simulink model "sf_multiword_fixpt"  (R2017b)
settings: Solver=FixedStepDiscrete  StartTime=0.0  StopTime=10.0  RelTol=1e-3  EnableMultiTasking=on
libraries: simulink x1
settings Model: Creator=The MathWorks, Inc.  LastModifiedBy=The MathWorks, Inc.
settings DataIOCC: LimitDataPoints=on  SaveFormat=Array
settings OptimizationCC: ExpressionDepthLimit=2147483647  LifeSpan=inf
settings DebuggingCC: UnderspecifiedInitializationDetection=Classic  MergeDetectMultiDrivingBlocksExec=none  FcnCallInpInsideContextMsg=warning  StateNameClashWarn=warning  StrictBusMsg=Warning  SFUnexpectedBacktrackingDiag=warning  SFNoUnconditionalDefaultTransitionDiag=warning  SFExecutionAtInitializationDiag=none
settings HardwareCC: ProdBitPerLong=64  ProdBitPerPointer=32  ProdBitPerSizeT=32  ProdBitPerPtrDiffT=32  ProdLargestAtomicFloat=None  ProdIntDivRoundTo=Undefined  ProdEndianess=Unspecified  ProdWordSize=32  ProdHWDeviceType=Generic->Custom  TargetHWDeviceType=32-bit Generic
settings ModelReferenceCC: PropagateSignalLabelsOutOfModel=off
settings SFSimCC: SimParseCustomCode=off
settings CodeAppCC: StateflowObjectComments=on
settings GRTTargetCC: TargetLangStandard=C89/C90 (ANSI)  GeneratePreprocessorConditionals=Disable all  CombineOutputUpdateFcns=off  GRTInterface=on
settings ConfigComp: CovMetricSettings=dw  CovHtmlReporting=on  CovSaveCumulativeToWorkspaceVar=on  CovSaveSingleToWorkspaceVar=on  CovExternalEMLEnable=off  CovSFcnEnable=off

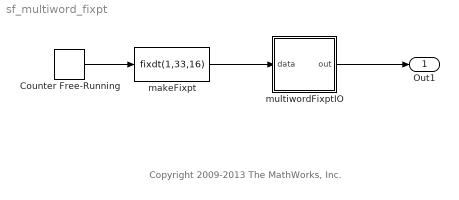
== system sf_multiword_fixpt ==
  note: Copyright 2009-2013 The MathWorks, Inc.
  Counter Free-Running : simulink/Sources/Counter Free-Running  NumBits=16  tsamp=-1
  makeFixpt : DataTypeConversion  OutDataTypeStr=fixdt(1,33,16)
  multiwordFixptIO : Stateflow chart  TreatAsAtomicUnit=on
  Out1 : Outport
  wires:
  multiwordFixptIO/1(out) -> Out1/1
  Counter Free-Running/1 -> makeFixpt/1
  makeFixpt/1 -> multiwordFixptIO/1(data)

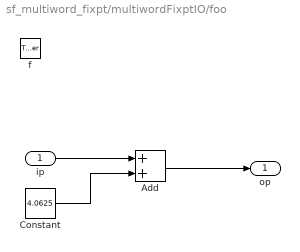
== system sf_multiword_fixpt/multiwordFixptIO/foo ==
  ip : Inport  OutDataTypeStr=fixdt(1,33,16)
  f : TriggerPort  TriggerType=function-call  VariantControl=(inherit)
      settings: CopyFcn=Stateflow.SLINSF.SimulinkMan.removeBlockPreDeleteFcn  PreDeleteFcn=Stateflow.SLINSF.SimulinkMan.unsafePredeleteFcn
  Add : Sum  OutDataTypeStr=fixdt(1,33,16)
  Constant : Constant  Value=4.0625  OutDataTypeStr=fixdt(1,16,4)
  op : Outport
  wires:
  ip/1 -> Add/1
  Constant/1 -> Add/2
  Add/1 -> op/1

== stateflow chart sf_multiword_fixpt/multiwordFixptIO ==
  state A
    du:
    out = foo(data);
  state op = foo(ip) [function]
  data: ip function_input fixdt(1,33,16); op function_output; data input fixdt(1,33,16); out output fixdt(1,33,16)
